simulink model "bilateral_control_wv"  (R2023a)
settings: Solver=VariableStepAuto  StartTime=0.0  StopTime=160  RelTol=1e-3
settings Model: Creator=UPM  LastModifiedBy=Josep

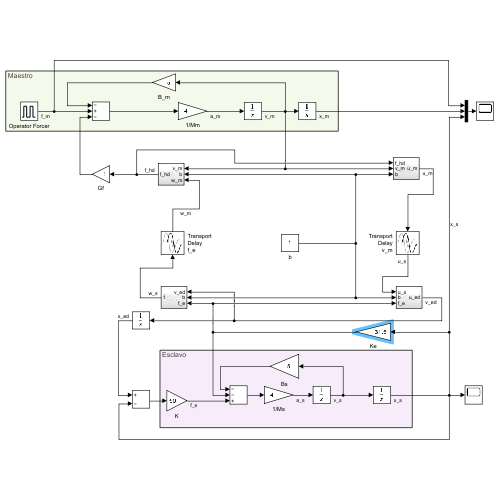
[thumbnail: Simulink's stored preview of the top-level diagram]
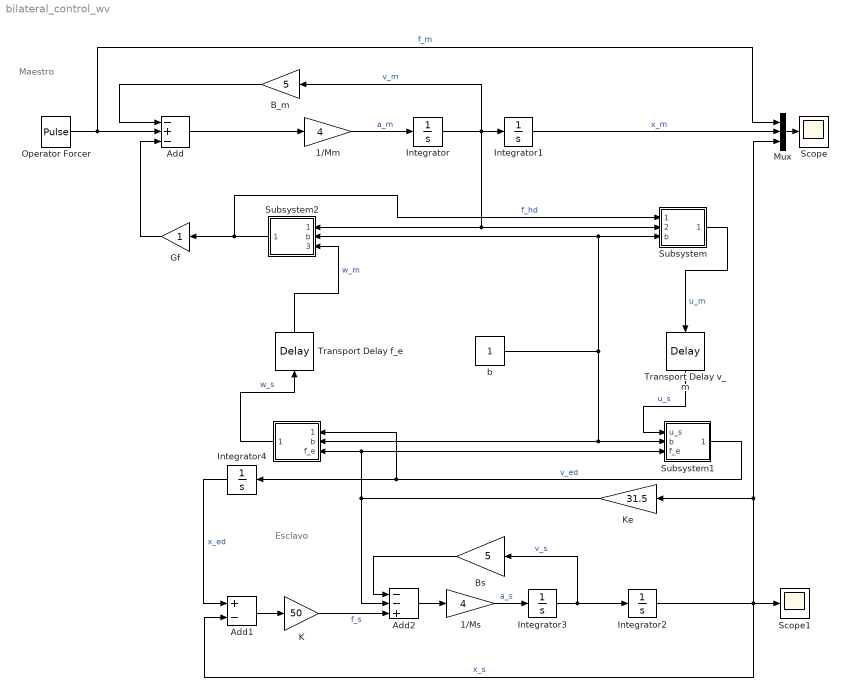
== system bilateral_control_wv ==
  note: Esclavo
  note: Maestro
  " " : Subsystem  Tag=v_m to u_m  Description=v_m to u_m
  1/Mm : Gain  Gain=4
  1/Ms : Gain  Gain=4
  Add : Sum  Inputs=-+-
  Add1 : Sum  Inputs=+-
  Add2 : Sum  Inputs=--+
  B_m : Gain  Gain=5
  Bs : Gain  Gain=5
  Gf : Gain
  Integrator{,1..4} (5 alike) : Integrator
  K : Gain  Gain=50
  Ke : Gain  Gain=31.5
  Mux : Mux  Inputs=3
  Operator Forcer : DiscretePulseGenerator  PulseType=Time based  Amplitude=4  Period=80  PulseWidth=50
  Scope : Scope
  Scope1 : Scope
  Subsystem : Subsystem  Tag=v_m to u_m  Description=v_m to u_m
  Subsystem1 : Subsystem  Tag=v_m to u_m  Description=v_m to u_m
  Subsystem2 : Subsystem  Tag=v_m to u_m  Description=v_m to u_m
  Transport Delay f_e : TransportDelay  DelayTime=0.05
  Transport Delay v_m : TransportDelay  DelayTime=0.05
  b : Constant  VectorParams1D=off
  wires:
  Integrator/1 -> Integrator1/1, Subsystem2/1(v_m), Subsystem/2(v_m), B_m/1  "v_m"
  Integrator3/1 -> Integrator2/1, Bs/1  "v_s"
  1/Mm/1 -> Integrator/1  "a_m"
  Integrator2/1 -> Add1/2, Ke/1, Mux/3, Scope1/1  "x_s"
  1/Ms/1 -> Integrator3/1  "a_s"
  Add1/1 -> K/1
  K/1 -> Add2/3  "f_s"
  Add2/1 -> 1/Ms/1
  Bs/1 -> Add2/1
  Add/1 -> 1/Mm/1
  Ke/1 -> Subsystem1/3(f_e), " "/3(f_e), Add2/2
  Operator Forcer/1 -> Mux/1, Add/2  "f_m"
  B_m/1 -> Add/1
  Gf/1 -> Add/3
  Integrator1/1 -> Mux/2  "x_m"
  Mux/1 -> Scope/1
  Subsystem/1(u_m) -> Transport Delay v_m/1  "u_m"
  b/1 -> Subsystem/3(b), Subsystem2/2(b), Subsystem1/2(b), " "/2(b)
  " "/1(Out1) -> Transport Delay f_e/1  "w_s"
  Transport Delay v_m/1 -> Subsystem1/1(u_s)  "u_s"
  Subsystem1/1(u_ed) -> " "/1(v_ed), Integrator4/1  "v_ed"
  Integrator4/1 -> Add1/1  "x_ed"
  Transport Delay f_e/1 -> Subsystem2/3(w_m)  "w_m"
  Subsystem2/1(f_hd) -> Subsystem/1(f_hd), Gf/1  "f_hd"

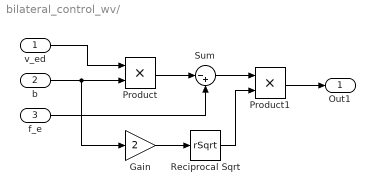
== system bilateral_control_wv/  ==
  v_ed : Inport
  b : Inport  Port=2
  f_e : Inport  Port=3
  Gain : Gain  Gain=2
  Product : Product
  Product1 : Product
  Reciprocal Sqrt : Sqrt  Operator=rSqrt
  Sum : Sum  Inputs=|-+
  Out1 : Outport
  wires:
  v_ed/1 -> Product/1
  Product/1 -> Sum/1
  f_e/1 -> Sum/2
  b/1 -> Product/2, Gain/1
  Gain/1 -> Reciprocal Sqrt/1
  Sum/1 -> Product1/1
  Reciprocal Sqrt/1 -> Product1/2
  Product1/1 -> Out1/1

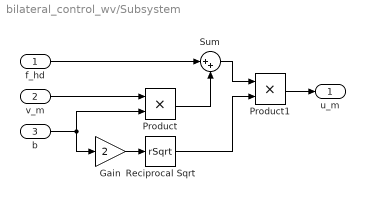
== system bilateral_control_wv/Subsystem ==
  f_hd : Inport
  v_m : Inport  Port=2
  b : Inport  Port=3
  Gain : Gain  Gain=2
  Product : Product
  Product1 : Product
  Reciprocal Sqrt : Sqrt  Operator=rSqrt
  Sum : Sum  Inputs=|++
  u_m : Outport
  wires:
  v_m/1 -> Product/1
  Product/1 -> Sum/2
  f_hd/1 -> Sum/1
  b/1 -> Product/2, Gain/1
  Gain/1 -> Reciprocal Sqrt/1
  Sum/1 -> Product1/1
  Reciprocal Sqrt/1 -> Product1/2
  Product1/1 -> u_m/1

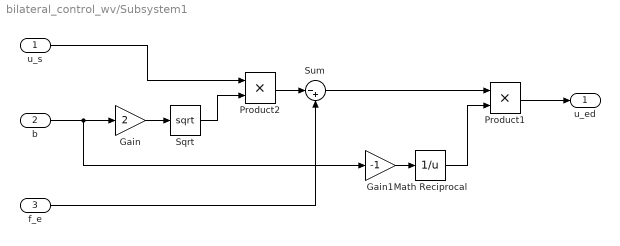
== system bilateral_control_wv/Subsystem1 ==
  u_s : Inport
  b : Inport  Port=2
  f_e : Inport  Port=3
  Gain : Gain  Gain=2
  Gain1 : Gain  Gain=-1
  Math Reciprocal : Math  Operator=reciprocal  SignedPower=on
  Product1 : Product
  Product2 : Product
  Sqrt : Sqrt
  Sum : Sum  Inputs=|-+
  u_ed : Outport
  wires:
  b/1 -> Gain1/1, Gain/1
  Gain/1 -> Sqrt/1
  Product2/1 -> Sum/1
  Sqrt/1 -> Product2/2
  u_s/1 -> Product2/1
  f_e/1 -> Sum/2
  Gain1/1 -> Math Reciprocal/1
  Math Reciprocal/1 -> Product1/2
  Sum/1 -> Product1/1
  Product1/1 -> u_ed/1

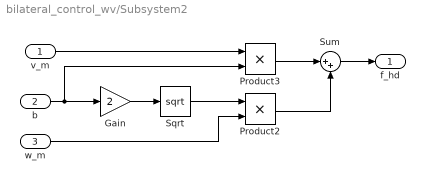
== system bilateral_control_wv/Subsystem2 ==
  v_m : Inport
  b : Inport  Port=2
  w_m : Inport  Port=3
  Gain : Gain  Gain=2
  Product2 : Product
  Product3 : Product
  Sqrt : Sqrt
  Sum : Sum  Inputs=|++
  f_hd : Outport
  wires:
  b/1 -> Product3/2, Gain/1
  Gain/1 -> Sqrt/1
  Sum/1 -> f_hd/1
  Sqrt/1 -> Product2/1
  w_m/1 -> Product2/2
  Product2/1 -> Sum/2
  v_m/1 -> Product3/1
  Product3/1 -> Sum/1
